simulink model "reg"  (R2024b)
settings: Solver=VariableStepAuto  StartTime=0.0  StopTime=tspan  RelTol=1e-3
values from neighbouring files (symbols this model uses):
  desr = [1 1.1]    [main.m]
  desr_val = 0.01    [main.m]
  Reg = ppc(dtf, poles)    [main.m]
undefined symbols (not defined in the file or in its folder): dspblkCoreblockFVToolHelper, dtf, gcbh

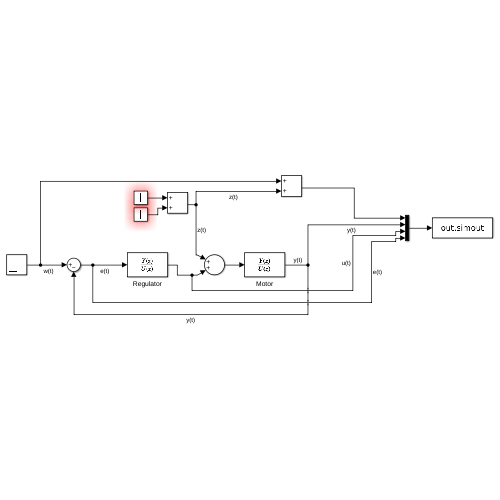
[thumbnail: Simulink's stored preview of the top-level diagram]
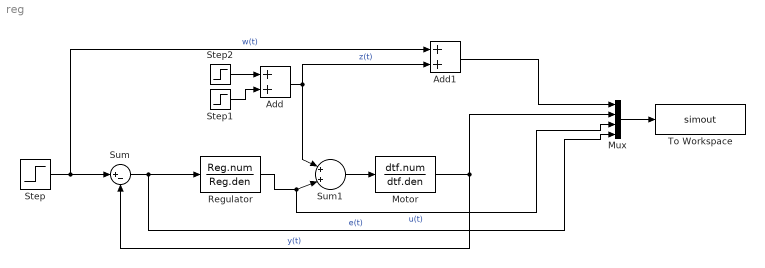
== system reg ==
  Add : Sum
  Add1 : Sum
  Motor : DiscreteTransferFcn  LoadFcn=dspblkCoreblockFVToolHelper(gcbh,'load');  Numerator=dtf.num  Denominator=dtf.den
      settings: CopyFcn=dspblkCoreblockFVToolHelper(gcbh,'copy');  DeleteFcn=dspblkCoreblockFVToolHelper(gcbh,'close');  ModelCloseFcn=dspblkCoreblockFVToolHelper(gcbh,'close');  PreSaveFcn=dspblkCoreblockFVToolHelper(gcbh,'presave');  PostSaveFcn=dspblkCoreblockFVToolHelper(gcbh,'postsave');  CloseFcn=dspblkCoreblockFVToolHelper(gcbh,'close');
  Mux : Mux
  Regulator : DiscreteTransferFcn  LoadFcn=dspblkCoreblockFVToolHelper(gcbh,'load');  Numerator=Reg.num  Denominator=Reg.den
      settings: CopyFcn=dspblkCoreblockFVToolHelper(gcbh,'copy');  DeleteFcn=dspblkCoreblockFVToolHelper(gcbh,'close');  ModelCloseFcn=dspblkCoreblockFVToolHelper(gcbh,'close');  PreSaveFcn=dspblkCoreblockFVToolHelper(gcbh,'presave');  PostSaveFcn=dspblkCoreblockFVToolHelper(gcbh,'postsave');  CloseFcn=dspblkCoreblockFVToolHelper(gcbh,'close');
  Step : Step  Time=0  SampleTime=0.08
  Step1 : Step  Time=desr(2)  After=-desr_val  SampleTime=0
  Step2 : Step  Time=desr(1)  After=desr_val  SampleTime=0
  Sum : Sum  Inputs=|+-
  Sum1 : Sum  Inputs=|++|
  To Workspace : ToWorkspace  VariableName=simout  SaveFormat=Timeseries  SampleTime=-1
  wires:
  Step/1 -> Add1/1, Sum/1  "w(t)"
  Sum/1 -> Mux/4, Regulator/1  "e(t)"
  Regulator/1 -> Mux/3, Sum1/2  "u(t)"
  Motor/1 -> Sum/2, Mux/2  "y(t)"
  Sum1/1 -> Motor/1
  Step1/1 -> Add/2
  Step2/1 -> Add/1
  Add/1 -> Add1/2, Sum1/1  "z(t)"
  Add1/1 -> Mux/1
  Mux/1 -> To Workspace/1
